simulink library "halout"  (R2021b)
settings: Solver=VariableStepAuto  StartTime=0.0  StopTime=10.0  RelTol=1e-3
undefined symbols (not defined in the file): C_TASK_5MS_S, FALSE, KHAL_CAN1FD1APS3E2E_flg, KHAL_CAN1FD1APS3TxReq_flg, KHAL_CAN1FD1VCU2E2E_flg, KHAL_CAN1FD1VCU2TxReq_flg, KHAL_CAN1FD1VCU3E2E_flg, KHAL_CAN1FD1VCU3TxReq_flg, KHAL_CAN1TxReq_flg, KHAL_CAN1VMCFCM1E2E_flg, KHAL_CAN1VMCFCM1TxReq_flg, KHAL_CAN2TxReq_flg, KHAL_CAN3FD3VCU1toNIDECTxReq_flg, KHAL_CAN3FD3VCU1TxReq_flg, KHAL_CAN3FD3VCU2E2E_flg, KHAL_CAN3FD3VCU2toNIDECE2E_flg, KHAL_CAN3FD3VCU2toNIDECTxReq_flg, KHAL_CAN3FD3VCU2TxReq_flg, KHAL_CAN3TxReq_flg, KHAL_CAN4FD4CE1000E2E_flg, KHAL_CAN4FD4CE1000TxReq_flg, KHAL_CAN4TxReq_flg, KHAL_CAN5TxReq_flg, KHAL_CAN6FD6APS3E2E_flg, KHAL_CAN6FD6APS3TxReq_flg, KHAL_CAN6FD6VCU2E2E_flg, KHAL_CAN6FD6VCU2TxReq_flg, KHAL_CAN6TxReq_flg, ONE_INT, TRUE, ZERO_INT
libraries: FVT_lib x500, simulink x235
(part 8 of 25)

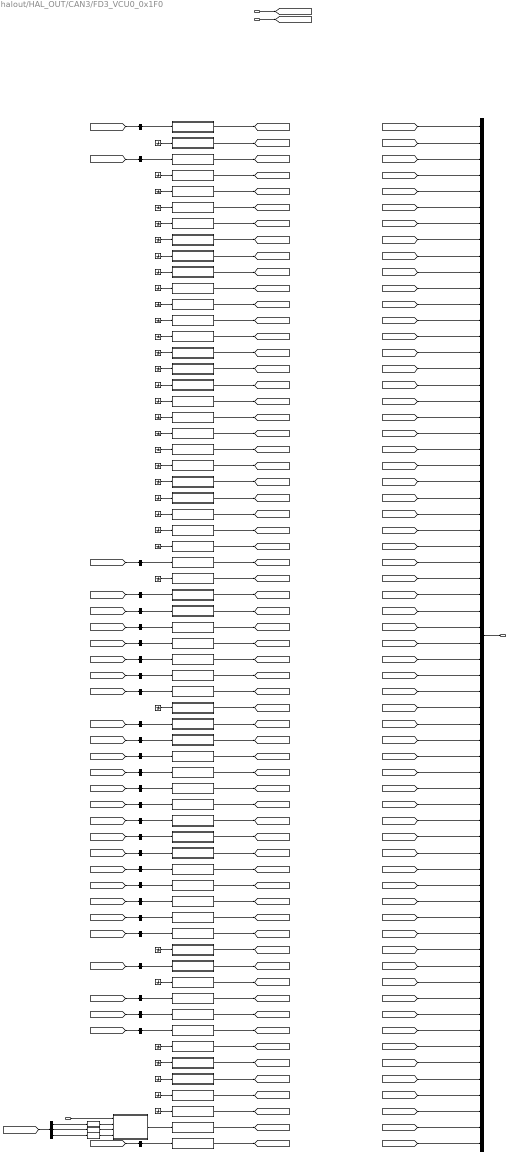
== system halout/HAL_OUT/CAN3/FD3_VCU0_0x1F0 ==
  BSCP_outputs : Inport  OutDataTypeStr=Bus: BSCP_outputs
  BOUTP_outputs : Inport  Port=2  OutDataTypeStr=Bus: BOUTP_outputs
  s8_AcoreReadyToSleep : Inport  Port=3
  Data Type Conversion : DataTypeConversion  OutDataTypeStr=uint8
  Data Type Conversion1 : DataTypeConversion  OutDataTypeStr=uint8
  Data Type Conversion2 : DataTypeConversion  OutDataTypeStr=uint8
  EVCCAplusPwrUpReq : Subsystem
  FDADC12VDet : Subsystem
  FDADC12VDetAvg : Subsystem
  FDCVCUActMaxSlideRateSta : Subsystem
  FDCVCUAllowMovThdOTASta : Subsystem
  FDCVCUDTCCarouselSta : Subsystem
  FDCVCUForcePCmd : Subsystem
  FDCVCUOTAPwrReqOFFChkSta : Subsystem
  FDCVCUOTAPwrReqStdChkSta : Subsystem
  FDCVCUPwrReqOTASta : Subsystem
  FDCVCURWDRDCActiveSta : Subsystem
  FDCVCURegenTqLimitEnSta : Subsystem
  FDCVCUSlideRegenLimTqSta : Subsystem
  FDCVCUVehActSpdSta : Subsystem
  FDCVCUVehMalfunLevelSta : Subsystem
  FDCVMCActStESCYawSta : Subsystem
  FDCVMCLongAccSta : Subsystem
  FUSIONCMM1 : Subsystem
  FUSIONCMM10 : Subsystem
  FUSIONCMM2 : Subsystem
  FUSIONCMM3 : Subsystem
  FUSIONCMM4 : Subsystem
  FUSIONCMM5 : Subsystem
  FUSIONCMM6 : Subsystem
  FUSIONCMM7 : Subsystem
  FUSIONCMM8 : Subsystem
  FUSIONCMM9 : Subsystem
  FrTqSource : Subsystem
  Ground{,1..33} (34 alike) : Ground
  HVRlyOpFail : Subsystem
  HVTHCMSysAvail : Subsystem
  LVBattChrgtimeAct : Subsystem
  LVBattVoltSta : Subsystem
  LVChrgHoldTAct : Subsystem
  LVSilentChrgLv : Subsystem
  LVSilentChrgReq : Subsystem
  LVSilentChrgSta : Subsystem
  MCUActDisFail : Subsystem
  PMMAllowECUSleep : Subsystem
  PmicBootReason : Subsystem
  PowerDownFault : Subsystem
  PowerDownState : Subsystem
  PowerUpFault : Subsystem
  PowerUpState : Subsystem
  PwrDownReq : Subsystem
  PwrStaConstraint : Subsystem
  PwrStaONTOIVIPopReq : Subsystem
  PwrStaONTOIVIPopT : Subsystem
  PwrStaSelect : Subsystem
  PwrStaTOSta : Subsystem
  PwrUpReq : Subsystem
  RrTqSource : Subsystem
  SchedChgTOSta : Subsystem
  SilentChkAllowSleep : Subsystem
  Subsystem : Subsystem
  SysAllowReadySta : Subsystem
  SysPwrSta : Subsystem
  TCountSta : Subsystem
  TimerAllowSleep : Subsystem
  VCUBrkSWSta : Subsystem
  VCUFLDoorSta : Subsystem
  VCUFRDoorSta : Subsystem
  VCURLDoorSta : Subsystem
  VCURRDoorSta : Subsystem
  VehHVPwrAvail4THCM : Subsystem
  WisrBootReason : Subsystem
  bus_creator : BusCreator  Inputs=64  OutDataTypeStr=Bus: DT_CAN3_SG_FD3_VCU0  NonVirtualBus=on
  bus_selector : BusSelector  OutputSignals=VOUTP_EvccAplusPwrUpReq_flg
  bus_selector1 : BusSelector  OutputSignals=VOUTP_FDADC12VDetAvg_mV
  bus_selector10 : BusSelector  OutputSignals=VOUTP_PMMAllowECUSleep_flg
  bus_selector11 : BusSelector  OutputSignals=VOUTP_PmicBootReason_enum
  bus_selector12 : BusSelector  OutputSignals=VOUTP_PowerDownFault_enum
  bus_selector13 : BusSelector  OutputSignals=VOUTP_PowerDownState_enum
  bus_selector14 : BusSelector  OutputSignals=VOUTP_PowerUpFault_enum
  bus_selector15 : BusSelector  OutputSignals=VOUTP_PowerUpState_enum
  bus_selector16 : BusSelector  OutputSignals=VOUTP_PwrDownReq_enum
  bus_selector17 : BusSelector  OutputSignals=VOUTP_PwrStaConstraint_enum
  bus_selector18 : BusSelector  OutputSignals=VOUTP_PwrStaONTOPopReq_flg
  bus_selector19 : BusSelector  OutputSignals=VOUTP_IVIPwrStaONTOPopT_s
  bus_selector2 : BusSelector  OutputSignals=VOUTP_TqSourceFr_enum
  bus_selector20 : BusSelector  OutputSignals=VOUTP_PwrStaSelect_enum
  bus_selector21 : BusSelector  OutputSignals=VOUTP_PwrStaTOSta_enum
  bus_selector22 : BusSelector  OutputSignals=VOUTP_PwrUpReq_enum
  bus_selector23 : BusSelector  OutputSignals=VOUTP_TqSourceRr_enum
  bus_selector24 : BusSelector  OutputSignals=VOUTP_SilentChkAllowSleep_flg
  bus_selector25 : BusSelector  OutputSignals=VOUTP_SysPowerMode_enum
  bus_selector26 : BusSelector  OutputSignals=VOUTP_TCountSta_enum
  bus_selector27 : BusSelector  OutputSignals=VOUTP_TimerAllowSleep_flg
  bus_selector28 : BusSelector  OutputSignals=VOUTP_CurrentNmState_enum,VOUTP_OTAPwrReqOFFChkSta_enum,VOUTP_OTAPwrReqStdChkSta_enum
  bus_selector29 : BusSelector  OutputSignals=VOUTP_WisrBootReason_raw32
  bus_selector3 : BusSelector  OutputSignals=VOUTP_HVTHCMSysAvail_enum
  bus_selector4 : BusSelector  OutputSignals=VOUTP_LVBattChrgTimeCnt_s
  bus_selector5 : BusSelector  OutputSignals=VOUTP_LVBattVoltSta_enum
  bus_selector6 : BusSelector  OutputSignals=VOUTP_LVChrgHoldTtimer_s
  bus_selector7 : BusSelector  OutputSignals=VOUTP_LVSilentChrgLv_enum
  bus_selector8 : BusSelector  OutputSignals=VOUTP_LVSilentChrgReq_flg
  bus_selector9 : BusSelector  OutputSignals=VOUTP_LVSilentChrgSta_enum
  FD3_VCU0 : Outport
  wires:
  BSCP_outputs/1 -> [BSCP_outputs]
  BOUTP_outputs/1 -> [BOUTP_outputs]
  [CAN3_EVCCAplusPwrUpReq] -> bus_creator/1  "CAN3_EVCCAplusPwrUpReq"
  [CAN3_FDADC12VDet] -> bus_creator/2  "CAN3_FDADC12VDet"
  [CAN3_FDADC12VDetAvg] -> bus_creator/3  "CAN3_FDADC12VDetAvg"
  [CAN3_FDC_VCU_ActMaxSlideRate_Sta] -> bus_creator/4  "CAN3_FDC_VCU_ActMaxSlideRate_Sta"
  [CAN3_FDC_VCU_AllowMovThd_OTA_Sta] -> bus_creator/5  "CAN3_FDC_VCU_AllowMovThd_OTA_Sta"
  [CAN3_FDC_VCU_DTCCarousel_Sta] -> bus_creator/6  "CAN3_FDC_VCU_DTCCarousel_Sta"
  [CAN3_FDC_VCU_ForceP_Cmd] -> bus_creator/7  "CAN3_FDC_VCU_ForceP_Cmd"
  [CAN3_FDC_VCU_OTAPwrReqOFFChk_Sta] -> bus_creator/8  "CAN3_FDC_VCU_OTAPwrReqOFFChk_Sta"
  [CAN3_FDC_VCU_OTAPwrReqStdChk_Sta] -> bus_creator/9  "CAN3_FDC_VCU_OTAPwrReqStdChk_Sta"
  [CAN3_FDC_VCU_PwrReq_OTA_Sta] -> bus_creator/10  "CAN3_FDC_VCU_PwrReq_OTA_Sta"
  [CAN3_FDC_VCU_RWDRDCActive_Sta] -> bus_creator/11  "CAN3_FDC_VCU_RWDRDCActive_Sta"
  [CAN3_FDC_VCU_RegenTqLimitEn_Sta] -> bus_creator/12  "CAN3_FDC_VCU_RegenTqLimitEn_Sta"
  [CAN3_FDC_VCU_SlideRegenLimTq_Sta] -> bus_creator/13  "CAN3_FDC_VCU_SlideRegenLimTq_Sta"
  [CAN3_FDC_VCU_VehActSpd_Sta] -> bus_creator/14  "CAN3_FDC_VCU_VehActSpd_Sta"
  [CAN3_FDC_VCU_VehMalfunLevel_Sta] -> bus_creator/15  "CAN3_FDC_VCU_VehMalfunLevel_Sta"
  [CAN3_FDC_VMC_ActStESCYaw_Sta] -> bus_creator/16  "CAN3_FDC_VMC_ActStESCYaw_Sta"
  [CAN3_FDC_VMC_LongAcc_Sta] -> bus_creator/17  "CAN3_FDC_VMC_LongAcc_Sta"
  [CAN3_FUSION_CMM1] -> bus_creator/18  "CAN3_FUSION_CMM1"
  [CAN3_FUSION_CMM10] -> bus_creator/19  "CAN3_FUSION_CMM10"
  [CAN3_FUSION_CMM2] -> bus_creator/20  "CAN3_FUSION_CMM2"
  [CAN3_FUSION_CMM3] -> bus_creator/21  "CAN3_FUSION_CMM3"
  [CAN3_FUSION_CMM4] -> bus_creator/22  "CAN3_FUSION_CMM4"
  [CAN3_FUSION_CMM5] -> bus_creator/23  "CAN3_FUSION_CMM5"
  [CAN3_FUSION_CMM6] -> bus_creator/24  "CAN3_FUSION_CMM6"
  [CAN3_FUSION_CMM7] -> bus_creator/25  "CAN3_FUSION_CMM7"
  [CAN3_FUSION_CMM8] -> bus_creator/26  "CAN3_FUSION_CMM8"
  [CAN3_FUSION_CMM9] -> bus_creator/27  "CAN3_FUSION_CMM9"
  [CAN3_Fr_TqSource] -> bus_creator/28  "CAN3_Fr_TqSource"
  [CAN3_HVRlyOpFail] -> bus_creator/29  "CAN3_HVRlyOpFail"
  [CAN3_HVTHCMSysAvail] -> bus_creator/30  "CAN3_HVTHCMSysAvail"
  [CAN3_LVBattChrgtimeAct] -> bus_creator/31  "CAN3_LVBattChrgtimeAct"
  [CAN3_LVBattVoltSta] -> bus_creator/32  "CAN3_LVBattVoltSta"
  [CAN3_LVChrgHoldTAct] -> bus_creator/33  "CAN3_LVChrgHoldTAct"
  [CAN3_LVSilentChrgLv] -> bus_creator/34  "CAN3_LVSilentChrgLv"
  [CAN3_LVSilentChrgReq] -> bus_creator/35  "CAN3_LVSilentChrgReq"
  [CAN3_LVSilentChrgSta] -> bus_creator/36  "CAN3_LVSilentChrgSta"
  [CAN3_MCUActDisFail] -> bus_creator/37  "CAN3_MCUActDisFail"
  [CAN3_PMMAllowECUSleep] -> bus_creator/38  "CAN3_PMMAllowECUSleep"
  [CAN3_PmicBootReason] -> bus_creator/39  "CAN3_PmicBootReason"
  [CAN3_PowerDownFault] -> bus_creator/40  "CAN3_PowerDownFault"
  [CAN3_PowerDownState] -> bus_creator/41  "CAN3_PowerDownState"
  [CAN3_PowerUpFault] -> bus_creator/42  "CAN3_PowerUpFault"
  [CAN3_PowerUpState] -> bus_creator/43  "CAN3_PowerUpState"
  [CAN3_PwrDownReq] -> bus_creator/44  "CAN3_PwrDownReq"
  [CAN3_PwrStaConstraint] -> bus_creator/45  "CAN3_PwrStaConstraint"
  [CAN3_PwrStaONTOIVIPopReq] -> bus_creator/46  "CAN3_PwrStaONTOIVIPopReq"
  [CAN3_PwrStaONTOIVIPopT] -> bus_creator/47  "CAN3_PwrStaONTOIVIPopT"
  [CAN3_PwrStaSelect] -> bus_creator/48  "CAN3_PwrStaSelect"
  [CAN3_PwrStaTOSta] -> bus_creator/49  "CAN3_PwrStaTOSta"
  [CAN3_PwrUpReq] -> bus_creator/50  "CAN3_PwrUpReq"
  [CAN3_Rr_TqSource] -> bus_creator/51  "CAN3_Rr_TqSource"
  [CAN3_SchedChgTOSta] -> bus_creator/52  "CAN3_SchedChgTOSta"
  [CAN3_SilentChkAllowSleep] -> bus_creator/53  "CAN3_SilentChkAllowSleep"
  [CAN3_SysAllowReadySta] -> bus_creator/54  "CAN3_SysAllowReadySta"
  [CAN3_SysPwrSta] -> bus_creator/55  "CAN3_SysPwrSta"
  [CAN3_TCountSta] -> bus_creator/56  "CAN3_TCountSta"
  [CAN3_TimerAllowSleep] -> bus_creator/57  "CAN3_TimerAllowSleep"
  [CAN3_VCUBrkSWSta] -> bus_creator/58  "CAN3_VCUBrkSWSta"
  [CAN3_VCUFLDoorSta] -> bus_creator/59  "CAN3_VCUFLDoorSta"
  [CAN3_VCUFRDoorSta] -> bus_creator/60  "CAN3_VCUFRDoorSta"
  [CAN3_VCURLDoorSta] -> bus_creator/61  "CAN3_VCURLDoorSta"
  [CAN3_VCURRDoorSta] -> bus_creator/62  "CAN3_VCURRDoorSta"
  [CAN3_VehHVPwrAvail4THCM] -> bus_creator/63  "CAN3_VehHVPwrAvail4THCM"
  [CAN3_WisrBootReason] -> bus_creator/64  "CAN3_WisrBootReason"
  bus_creator/1 -> FD3_VCU0/1
  EVCCAplusPwrUpReq/1(CAN3_EVCCAplusPwrUpReq) -> [CAN3_EVCCAplusPwrUpReq]
  FDADC12VDet/1(CAN3_FDADC12VDet) -> [CAN3_FDADC12VDet]
  FDADC12VDetAvg/1(CAN3_FDADC12VDetAvg) -> [CAN3_FDADC12VDetAvg]
  FDCVCUActMaxSlideRateSta/1(CAN3_FDC_VCU_ActMaxSlideRate_Sta) -> [CAN3_FDC_VCU_ActMaxSlideRate_Sta]
  FDCVCUAllowMovThdOTASta/1(CAN3_FDC_VCU_AllowMovThd_OTA_Sta) -> [CAN3_FDC_VCU_AllowMovThd_OTA_Sta]
  FDCVCUDTCCarouselSta/1(CAN3_FDC_VCU_DTCCarousel_Sta) -> [CAN3_FDC_VCU_DTCCarousel_Sta]
  FDCVCUForcePCmd/1(CAN3_FDC_VCU_ForceP_Cmd) -> [CAN3_FDC_VCU_ForceP_Cmd]
  FDCVCUOTAPwrReqOFFChkSta/1(CAN3_FDC_VCU_OTAPwrReqOFFChk_Sta) -> [CAN3_FDC_VCU_OTAPwrReqOFFChk_Sta]
  FDCVCUOTAPwrReqStdChkSta/1(CAN3_FDC_VCU_OTAPwrReqStdChk_Sta) -> [CAN3_FDC_VCU_OTAPwrReqStdChk_Sta]
  FDCVCUPwrReqOTASta/1(CAN3_FDC_VCU_PwrReq_OTA_Sta) -> [CAN3_FDC_VCU_PwrReq_OTA_Sta]
  FDCVCURWDRDCActiveSta/1(CAN3_FDC_VCU_RWDRDCActive_Sta) -> [CAN3_FDC_VCU_RWDRDCActive_Sta]
  FDCVCURegenTqLimitEnSta/1(CAN3_FDC_VCU_RegenTqLimitEn_Sta) -> [CAN3_FDC_VCU_RegenTqLimitEn_Sta]
  FDCVCUSlideRegenLimTqSta/1(CAN3_FDC_VCU_SlideRegenLimTq_Sta) -> [CAN3_FDC_VCU_SlideRegenLimTq_Sta]
  FDCVCUVehActSpdSta/1(CAN3_FDC_VCU_VehActSpd_Sta) -> [CAN3_FDC_VCU_VehActSpd_Sta]
  FDCVCUVehMalfunLevelSta/1(CAN3_FDC_VCU_VehMalfunLevel_Sta) -> [CAN3_FDC_VCU_VehMalfunLevel_Sta]
  FDCVMCActStESCYawSta/1(CAN3_FDC_VMC_ActStESCYaw_Sta) -> [CAN3_FDC_VMC_ActStESCYaw_Sta]
  FDCVMCLongAccSta/1(CAN3_FDC_VMC_LongAcc_Sta) -> [CAN3_FDC_VMC_LongAcc_Sta]
  FUSIONCMM1/1(CAN3_FUSION_CMM1) -> [CAN3_FUSION_CMM1]
  FUSIONCMM10/1(CAN3_FUSION_CMM10) -> [CAN3_FUSION_CMM10]
  FUSIONCMM2/1(CAN3_FUSION_CMM2) -> [CAN3_FUSION_CMM2]
  FUSIONCMM3/1(CAN3_FUSION_CMM3) -> [CAN3_FUSION_CMM3]
  FUSIONCMM4/1(CAN3_FUSION_CMM4) -> [CAN3_FUSION_CMM4]
  FUSIONCMM5/1(CAN3_FUSION_CMM5) -> [CAN3_FUSION_CMM5]
  FUSIONCMM6/1(CAN3_FUSION_CMM6) -> [CAN3_FUSION_CMM6]
  FUSIONCMM7/1(CAN3_FUSION_CMM7) -> [CAN3_FUSION_CMM7]
  FUSIONCMM8/1(CAN3_FUSION_CMM8) -> [CAN3_FUSION_CMM8]
  FUSIONCMM9/1(CAN3_FUSION_CMM9) -> [CAN3_FUSION_CMM9]
  FrTqSource/1(CAN3_Fr_TqSource) -> [CAN3_Fr_TqSource]
  HVRlyOpFail/1(CAN3_HVRlyOpFail) -> [CAN3_HVRlyOpFail]
  HVTHCMSysAvail/1(CAN3_HVTHCMSysAvail) -> [CAN3_HVTHCMSysAvail]
  LVBattChrgtimeAct/1(CAN3_LVBattChrgtimeAct) -> [CAN3_LVBattChrgtimeAct]
  LVBattVoltSta/1(CAN3_LVBattVoltSta) -> [CAN3_LVBattVoltSta]
  LVChrgHoldTAct/1(CAN3_LVChrgHoldTAct) -> [CAN3_LVChrgHoldTAct]
  LVSilentChrgLv/1(CAN3_LVSilentChrgLv) -> [CAN3_LVSilentChrgLv]
  LVSilentChrgReq/1(CAN3_LVSilentChrgReq) -> [CAN3_LVSilentChrgReq]
  LVSilentChrgSta/1(CAN3_LVSilentChrgSta) -> [CAN3_LVSilentChrgSta]
  MCUActDisFail/1(CAN3_MCUActDisFail) -> [CAN3_MCUActDisFail]
  PMMAllowECUSleep/1(CAN3_PMMAllowECUSleep) -> [CAN3_PMMAllowECUSleep]
  PmicBootReason/1(CAN3_PmicBootReason) -> [CAN3_PmicBootReason]
  PowerDownFault/1(CAN3_PowerDownFault) -> [CAN3_PowerDownFault]
  PowerDownState/1(CAN3_PowerDownState) -> [CAN3_PowerDownState]
  PowerUpFault/1(CAN3_PowerUpFault) -> [CAN3_PowerUpFault]
  PowerUpState/1(CAN3_PowerUpState) -> [CAN3_PowerUpState]
  PwrDownReq/1(CAN3_PwrDownReq) -> [CAN3_PwrDownReq]
  PwrStaConstraint/1(CAN3_PwrStaConstraint) -> [CAN3_PwrStaConstraint]
  PwrStaONTOIVIPopReq/1(CAN3_PwrStaONTOIVIPopReq) -> [CAN3_PwrStaONTOIVIPopReq]
  PwrStaONTOIVIPopT/1(CAN3_PwrStaONTOIVIPopT) -> [CAN3_PwrStaONTOIVIPopT]
  PwrStaSelect/1(CAN3_PwrStaSelect) -> [CAN3_PwrStaSelect]
  PwrStaTOSta/1(CAN3_PwrStaTOSta) -> [CAN3_PwrStaTOSta]
  PwrUpReq/1(CAN3_PwrUpReq) -> [CAN3_PwrUpReq]
  RrTqSource/1(CAN3_Rr_TqSource) -> [CAN3_Rr_TqSource]
  SchedChgTOSta/1(CAN3_SchedChgTOSta) -> [CAN3_SchedChgTOSta]
  SilentChkAllowSleep/1(CAN3_SilentChkAllowSleep) -> [CAN3_SilentChkAllowSleep]
  SysAllowReadySta/1(CAN3_SysAllowReadySta) -> [CAN3_SysAllowReadySta]
  SysPwrSta/1(CAN3_SysPwrSta) -> [CAN3_SysPwrSta]
  TCountSta/1(CAN3_TCountSta) -> [CAN3_TCountSta]
  TimerAllowSleep/1(CAN3_TimerAllowSleep) -> [CAN3_TimerAllowSleep]
  VCUBrkSWSta/1(CAN3_VCUBrkSWSta) -> [CAN3_VCUBrkSWSta]
  VCUFLDoorSta/1(CAN3_VCUFLDoorSta) -> [CAN3_VCUFLDoorSta]
  VCUFRDoorSta/1(CAN3_VCUFRDoorSta) -> [CAN3_VCUFRDoorSta]
  VCURLDoorSta/1(CAN3_VCURLDoorSta) -> [CAN3_VCURLDoorSta]
  VCURRDoorSta/1(CAN3_VCURRDoorSta) -> [CAN3_VCURRDoorSta]
  VehHVPwrAvail4THCM/1(CAN3_VehHVPwrAvail4THCM) -> [CAN3_VehHVPwrAvail4THCM]
  WisrBootReason/1(CAN3_WisrBootReason) -> [CAN3_WisrBootReason]
  bus_selector/1 -> EVCCAplusPwrUpReq/1(EVCCAplusPwrUpReq)  "<VOUTP_EvccAplusPwrUpReq_flg>"
  [BOUTP_outputs] -> bus_selector/1
  Ground/1 -> FDADC12VDet/1(FDADC12VDet)
  bus_selector1/1 -> FDADC12VDetAvg/1(FDADC12VDetAvg)  "<VOUTP_FDADC12VDetAvg_mV>"
  [BOUTP_outputs] -> bus_selector1/1
  Ground1/1 -> FDCVCUActMaxSlideRateSta/1(FDCVCUActMaxSlideRateSta)
  Ground2/1 -> FDCVCUAllowMovThdOTASta/1(FDCVCUAllowMovThdOTASta)
  Ground3/1 -> FDCVCUDTCCarouselSta/1(FDCVCUDTCCarouselSta)
  Ground4/1 -> FDCVCUForcePCmd/1(FDCVCUForcePCmd)
  Ground5/1 -> FDCVCUOTAPwrReqOFFChkSta/1(FDCVCUOTAPwrReqOFFChkSta)
  Ground6/1 -> FDCVCUOTAPwrReqStdChkSta/1(FDCVCUOTAPwrReqStdChkSta)
  Ground7/1 -> FDCVCUPwrReqOTASta/1(FDCVCUPwrReqOTASta)
  Ground8/1 -> FDCVCURWDRDCActiveSta/1(FDCVCURWDRDCActiveSta)
  Ground9/1 -> FDCVCURegenTqLimitEnSta/1(FDCVCURegenTqLimitEnSta)
  Ground10/1 -> FDCVCUSlideRegenLimTqSta/1(FDCVCUSlideRegenLimTqSta)
  Ground11/1 -> FDCVCUVehActSpdSta/1(FDCVCUVehActSpdSta)
  Ground12/1 -> FDCVCUVehMalfunLevelSta/1(FDCVCUVehMalfunLevelSta)
  Ground13/1 -> FDCVMCActStESCYawSta/1(FDCVMCActStESCYawSta)
  Ground14/1 -> FDCVMCLongAccSta/1(FDCVMCLongAccSta)
  Ground15/1 -> FUSIONCMM1/1(FUSIONCMM1)
  Ground16/1 -> FUSIONCMM10/1(FUSIONCMM10)
  Ground17/1 -> FUSIONCMM2/1(FUSIONCMM2)
  Ground18/1 -> FUSIONCMM3/1(FUSIONCMM3)
  Ground19/1 -> FUSIONCMM4/1(FUSIONCMM4)
  Ground20/1 -> FUSIONCMM5/1(FUSIONCMM5)
  Ground21/1 -> FUSIONCMM6/1(FUSIONCMM6)
  Ground22/1 -> FUSIONCMM7/1(FUSIONCMM7)
  Ground23/1 -> FUSIONCMM8/1(FUSIONCMM8)
  Ground24/1 -> FUSIONCMM9/1(FUSIONCMM9)
  bus_selector2/1 -> FrTqSource/1(FrTqSource)  "<VOUTP_TqSourceFr_enum>"
  [BOUTP_outputs] -> bus_selector2/1
  Ground25/1 -> HVRlyOpFail/1(HVRlyOpFail)
  bus_selector3/1 -> HVTHCMSysAvail/1(HVTHCMSysAvail)  "<VOUTP_HVTHCMSysAvail_enum>"
  [BOUTP_outputs] -> bus_selector3/1
  bus_selector4/1 -> LVBattChrgtimeAct/1(LVBattChrgtimeAct)  "<VOUTP_LVBattChrgTimeCnt_s>"
  [BOUTP_outputs] -> bus_selector4/1
  bus_selector5/1 -> LVBattVoltSta/1(LVBattVoltSta)  "<VOUTP_LVBattVoltSta_enum>"
  [BOUTP_outputs] -> bus_selector5/1
  bus_selector6/1 -> LVChrgHoldTAct/1(LVChrgHoldTAct)  "<VOUTP_LVChrgHoldTtimer_s>"
  [BOUTP_outputs] -> bus_selector6/1
  bus_selector7/1 -> LVSilentChrgLv/1(LVSilentChrgLv)  "<VOUTP_LVSilentChrgLv_enum>"
  [BOUTP_outputs] -> bus_selector7/1
  bus_selector8/1 -> LVSilentChrgReq/1(LVSilentChrgReq)  "<VOUTP_LVSilentChrgReq_flg>"
  [BOUTP_outputs] -> bus_selector8/1
  bus_selector9/1 -> LVSilentChrgSta/1(LVSilentChrgSta)  "<VOUTP_LVSilentChrgSta_enum>"
  [BOUTP_outputs] -> bus_selector9/1
  Ground26/1 -> MCUActDisFail/1(MCUActDisFail)
  bus_selector10/1 -> PMMAllowECUSleep/1(PMMAllowECUSleep)  "<VOUTP_PMMAllowECUSleep_flg>"
  [BOUTP_outputs] -> bus_selector10/1
  bus_selector11/1 -> PmicBootReason/1(PmicBootReason)  "<VOUTP_PmicBootReason_enum>"
  [BOUTP_outputs] -> bus_selector11/1
  bus_selector12/1 -> PowerDownFault/1(PowerDownFault)  "<VOUTP_PowerDownFault_enum>"
  [BOUTP_outputs] -> bus_selector12/1
  bus_selector13/1 -> PowerDownState/1(PowerDownState)  "<VOUTP_PowerDownState_enum>"
  [BOUTP_outputs] -> bus_selector13/1
  bus_selector14/1 -> PowerUpFault/1(PowerUpFault)  "<VOUTP_PowerUpFault_enum>"
  [BOUTP_outputs] -> bus_selector14/1
  bus_selector15/1 -> PowerUpState/1(PowerUpState)  "<VOUTP_PowerUpState_enum>"
  [BOUTP_outputs] -> bus_selector15/1
  bus_selector16/1 -> PwrDownReq/1(PwrDownReq)  "<VOUTP_PwrDownReq_enum>"
  [BOUTP_outputs] -> bus_selector16/1
  bus_selector17/1 -> PwrStaConstraint/1(PwrStaConstraint)  "<VOUTP_PwrStaConstraint_enum>"
  [BOUTP_outputs] -> bus_selector17/1
  bus_selector18/1 -> PwrStaONTOIVIPopReq/1(PwrStaONTOIVIPopReq)  "<VOUTP_PwrStaONTOPopReq_flg>"
  [BOUTP_outputs] -> bus_selector18/1
  bus_selector19/1 -> PwrStaONTOIVIPopT/1(PwrStaONTOIVIPopT)  "<VOUTP_IVIPwrStaONTOPopT_s>"
  [BOUTP_outputs] -> bus_selector19/1
  bus_selector20/1 -> PwrStaSelect/1(PwrStaSelect)  "<VOUTP_PwrStaSelect_enum>"
  [BOUTP_outputs] -> bus_selector20/1
  bus_selector21/1 -> PwrStaTOSta/1(PwrStaTOSta)  "<VOUTP_PwrStaTOSta_enum>"
  [BOUTP_outputs] -> bus_selector21/1
  bus_selector22/1 -> PwrUpReq/1(PwrUpReq)  "<VOUTP_PwrUpReq_enum>"
  [BOUTP_outputs] -> bus_selector22/1
  bus_selector23/1 -> RrTqSource/1(RrTqSource)  "<VOUTP_TqSourceRr_enum>"
  [BOUTP_outputs] -> bus_selector23/1
  Ground27/1 -> SchedChgTOSta/1(SchedChgTOSta)
  bus_selector24/1 -> SilentChkAllowSleep/1(SilentChkAllowSleep)  "<VOUTP_SilentChkAllowSleep_flg>"
  [BOUTP_outputs] -> bus_selector24/1
  Ground28/1 -> SysAllowReadySta/1(SysAllowReadySta)
  bus_selector25/1 -> SysPwrSta/1(SysPwrSta)  "<VOUTP_SysPowerMode_enum>"
  [BOUTP_outputs] -> bus_selector25/1
  bus_selector26/1 -> TCountSta/1(TCountSta)  "<VOUTP_TCountSta_enum>"
  [BOUTP_outputs] -> bus_selector26/1
  bus_selector27/1 -> TimerAllowSleep/1(TimerAllowSleep)  "<VOUTP_TimerAllowSleep_flg>"
  [BOUTP_outputs] -> bus_selector27/1
  Ground29/1 -> VCUBrkSWSta/1(VCUBrkSWSta)
  Ground30/1 -> VCUFLDoorSta/1(VCUFLDoorSta)
  Ground31/1 -> VCUFRDoorSta/1(VCUFRDoorSta)
  Ground32/1 -> VCURLDoorSta/1(VCURLDoorSta)
  Ground33/1 -> VCURRDoorSta/1(VCURRDoorSta)
  bus_selector29/1 -> WisrBootReason/1(WisrBootReason)  "<VOUTP_WisrBootReason_raw32>"
  [BOUTP_outputs] -> bus_selector29/1
  Subsystem/1(VehHVPwrAvail4THCM) -> VehHVPwrAvail4THCM/1(VehHVPwrAvail4THCM)
  bus_selector28/2 -> Data Type Conversion1/1  "<VOUTP_OTAPwrReqOFFChkSta_enum>"
  Data Type Conversion2/1 -> Subsystem/4(VOUTP_OTAPwrReqStdChkSta_enum)
  bus_selector28/1 -> Data Type Conversion/1  "<VOUTP_CurrentNmState_enum>"
  bus_selector28/3 -> Data Type Conversion2/1  "<VOUTP_OTAPwrReqStdChkSta_enum>"
  Data Type Conversion1/1 -> Subsystem/3(VOUTP_OTAPwrReqOFFChkSta_enum)
  Data Type Conversion/1 -> Subsystem/2(VOUTP_CurrentNmState_enum)
  [BOUTP_outputs] -> bus_selector28/1
  s8_AcoreReadyToSleep/1 -> Subsystem/1(s8_AcoreReadyToSleep)

== system halout/HAL_OUT/CAN3/FD3_VCU1_0x115 ==
  BSCP_outputs : Inport  OutDataTypeStr=Bus: BSCP_outputs
  BOUTP_outputs : Inport  Port=2  OutDataTypeStr=Bus: BOUTP_outputs
  ActiveDischReq : Subsystem
  CSVCU1 : Subsystem
  CoastDwModeStaChk : Subsystem
  DCDCEnaReq : Subsystem
  DCDCVoltSetpoint : Subsystem
  DemoModeStaChk : Subsystem
  DrSeatSta : Subsystem
  DynoModeStaChk : Subsystem
  Ground{,1..6} (7 alike) : Ground
  HVBatCnctReq : Subsystem
  HVSysReadyToCharge : Subsystem
  LVChrgFuncStaChk : Subsystem
  MSACrlSta : Subsystem
  PButtonSta : Subsystem
  PrkReq : Subsystem
  PrkReqValid : Subsystem
  PwrSta : Subsystem
  RCVCU1 : Subsystem
  ShiftGearPosn : Subsystem
  bus_creator : BusCreator  Inputs=18  OutDataTypeStr=Bus: DT_CAN3_SG_FD3_VCU1  NonVirtualBus=on
  bus_selector : BusSelector  OutputSignals=VOUTP_ActiveDischargeReq_flg
  bus_selector1 : BusSelector  OutputSignals=VOUTP_DCDCEnaReq_flg
  bus_selector10 : BusSelector  OutputSignals=VOUTP_ShiftGearPosn_enum
  bus_selector2 : BusSelector  OutputSignals=VOUTP_DCDCVoltSetpoint_V
  bus_selector3 : BusSelector  OutputSignals=VOUTP_DrSeatSta_enum
  bus_selector4 : BusSelector  OutputSignals=VOUTP_HVBatCnctReq_flg
  bus_selector5 : BusSelector  OutputSignals=VOUTP_HVSysReadyToCharge_enum
  bus_selector6 : BusSelector  OutputSignals=VOUTP_MSACtrlSta_enum
  bus_selector7 : BusSelector  OutputSignals=VOUTP_PButtonSta_enum
  bus_selector8 : BusSelector  OutputSignals=VOUTP_ActParkRequest_flg
  bus_selector9 : BusSelector  OutputSignals=VOUTP_PowerSta_enum
  FD3_VCU1 : Outport
  wires:
  BSCP_outputs/1 -> [BSCP_outputs]
  BOUTP_outputs/1 -> [BOUTP_outputs]
  [CAN3_ActiveDischReq] -> bus_creator/1  "CAN3_ActiveDischReq"
  [CAN3_CS_VCU1] -> bus_creator/2  "CAN3_CS_VCU1"
  [CAN3_CoastDwModeStaChk] -> bus_creator/3  "CAN3_CoastDwModeStaChk"
  [CAN3_DCDCEnaReq] -> bus_creator/4  "CAN3_DCDCEnaReq"
  [CAN3_DCDCVoltSetpoint] -> bus_creator/5  "CAN3_DCDCVoltSetpoint"
  [CAN3_DemoModeStaChk] -> bus_creator/6  "CAN3_DemoModeStaChk"
  [CAN3_Dr_SeatSta] -> bus_creator/7  "CAN3_Dr_SeatSta"
  [CAN3_DynoModeStaChk] -> bus_creator/8  "CAN3_DynoModeStaChk"
  [CAN3_HVBatCnctReq] -> bus_creator/9  "CAN3_HVBatCnctReq"
  [CAN3_HVSysReadyToCharge] -> bus_creator/10  "CAN3_HVSysReadyToCharge"
  [CAN3_LVChrgFuncStaChk] -> bus_creator/11  "CAN3_LVChrgFuncStaChk"
  [CAN3_MSA_Crl_Sta] -> bus_creator/12  "CAN3_MSA_Crl_Sta"
  [CAN3_P_Button_Sta] -> bus_creator/13  "CAN3_P_Button_Sta"
  [CAN3_PrkReq] -> bus_creator/14  "CAN3_PrkReq"
  [CAN3_PrkReqValid] -> bus_creator/15  "CAN3_PrkReqValid"
  [CAN3_PwrSta] -> bus_creator/16  "CAN3_PwrSta"
  [CAN3_RC_VCU1] -> bus_creator/17  "CAN3_RC_VCU1"
  [CAN3_ShiftGearPosn] -> bus_creator/18  "CAN3_ShiftGearPosn"
  bus_creator/1 -> FD3_VCU1/1
  ActiveDischReq/1(CAN3_ActiveDischReq) -> [CAN3_ActiveDischReq]
  CSVCU1/1(CAN3_CS_VCU1) -> [CAN3_CS_VCU1]
  CoastDwModeStaChk/1(CAN3_CoastDwModeStaChk) -> [CAN3_CoastDwModeStaChk]
  DCDCEnaReq/1(CAN3_DCDCEnaReq) -> [CAN3_DCDCEnaReq]
  DCDCVoltSetpoint/1(CAN3_DCDCVoltSetpoint) -> [CAN3_DCDCVoltSetpoint]
  DemoModeStaChk/1(CAN3_DemoModeStaChk) -> [CAN3_DemoModeStaChk]
  DrSeatSta/1(CAN3_Dr_SeatSta) -> [CAN3_Dr_SeatSta]
  DynoModeStaChk/1(CAN3_DynoModeStaChk) -> [CAN3_DynoModeStaChk]
  HVBatCnctReq/1(CAN3_HVBatCnctReq) -> [CAN3_HVBatCnctReq]
  HVSysReadyToCharge/1(CAN3_HVSysReadyToCharge) -> [CAN3_HVSysReadyToCharge]
  LVChrgFuncStaChk/1(CAN3_LVChrgFuncStaChk) -> [CAN3_LVChrgFuncStaChk]
  MSACrlSta/1(CAN3_MSA_Crl_Sta) -> [CAN3_MSA_Crl_Sta]
  PButtonSta/1(CAN3_P_Button_Sta) -> [CAN3_P_Button_Sta]
  PrkReq/1(CAN3_PrkReq) -> [CAN3_PrkReq]
  PrkReqValid/1(CAN3_PrkReqValid) -> [CAN3_PrkReqValid]
  PwrSta/1(CAN3_PwrSta) -> [CAN3_PwrSta]
  RCVCU1/1(CAN3_RC_VCU1) -> [CAN3_RC_VCU1]
  ShiftGearPosn/1(CAN3_ShiftGearPosn) -> [CAN3_ShiftGearPosn]
  bus_selector/1 -> ActiveDischReq/1(ActiveDischReq)  "<VOUTP_ActiveDischargeReq_flg>"
  [BOUTP_outputs] -> bus_selector/1
  Ground/1 -> CSVCU1/1(CSVCU1)
  Ground1/1 -> CoastDwModeStaChk/1(CoastDwModeStaChk)
  bus_selector1/1 -> DCDCEnaReq/1(DCDCEnaReq)  "<VOUTP_DCDCEnaReq_flg>"
  [BOUTP_outputs] -> bus_selector1/1
  bus_selector2/1 -> DCDCVoltSetpoint/1(DCDCVoltSetpoint)  "<VOUTP_DCDCVoltSetpoint_V>"
  [BOUTP_outputs] -> bus_selector2/1
  Ground2/1 -> DemoModeStaChk/1(DemoModeStaChk)
  bus_selector3/1 -> DrSeatSta/1(DrSeatSta)  "<VOUTP_DrSeatSta_enum>"
  [BOUTP_outputs] -> bus_selector3/1
  Ground3/1 -> DynoModeStaChk/1(DynoModeStaChk)
  bus_selector4/1 -> HVBatCnctReq/1(HVBatCnctReq)  "<VOUTP_HVBatCnctReq_flg>"
  [BOUTP_outputs] -> bus_selector4/1
  bus_selector5/1 -> HVSysReadyToCharge/1(HVSysReadyToCharge)  "<VOUTP_HVSysReadyToCharge_enum>"
  [BOUTP_outputs] -> bus_selector5/1
  Ground4/1 -> LVChrgFuncStaChk/1(LVChrgFuncStaChk)
  bus_selector6/1 -> MSACrlSta/1(MSACrlSta)  "<VOUTP_MSACtrlSta_enum>"
  [BOUTP_outputs] -> bus_selector6/1
  bus_selector7/1 -> PButtonSta/1(PButtonSta)  "<VOUTP_PButtonSta_enum>"
  [BOUTP_outputs] -> bus_selector7/1
  bus_selector8/1 -> PrkReq/1(PrkReq)  "<VOUTP_ActParkRequest_flg>"
  [BOUTP_outputs] -> bus_selector8/1
  Ground5/1 -> PrkReqValid/1(PrkReqValid)
  bus_selector9/1 -> PwrSta/1(PwrSta)  "<VOUTP_PowerSta_enum>"
  [BOUTP_outputs] -> bus_selector9/1
  Ground6/1 -> RCVCU1/1(RCVCU1)
  bus_selector10/1 -> ShiftGearPosn/1(ShiftGearPosn)  "<VOUTP_ShiftGearPosn_enum>"
  [BOUTP_outputs] -> bus_selector10/1

== system halout/HAL_OUT/CAN3/FD3_VCU1_Tx ==
  TxReq : Inport
  BSCP_outputs : Inport  Port=2  OutDataTypeStr=Bus: BSCP_outputs
  BOUTP_outputs : Inport  Port=3  OutDataTypeStr=Bus: BOUTP_outputs
  Chart : Stateflow chart  TreatAsAtomicUnit=on
  Constant : Constant  Value=C_TASK_5MS_S
  Constant3 : Constant  Value=CycleTime
  Data Type Conversion : DataTypeConversion  OutDataTypeStr=uint16
  Data Type Conversion1 : DataTypeConversion  OutDataTypeStr=uint8
  Divide : Product  Inputs=*/
  Gain : Gain  Gain=0.001
  Ground{,1..6} (7 alike) : Ground
  OR : Logic  Operator=OR  Inputs=18  AllPortsSameDT=off  OutDataTypeStr=boolean
  bus_selector : BusSelector  OutputSignals=VOUTP_ActiveDischargeReq_flg
  bus_selector1 : BusSelector  OutputSignals=VOUTP_DCDCEnaReq_flg
  bus_selector10 : BusSelector  OutputSignals=VOUTP_ShiftGearPosn_enum
  bus_selector2 : BusSelector  OutputSignals=VOUTP_DCDCVoltSetpoint_V
  bus_selector3 : BusSelector  OutputSignals=VOUTP_DrSeatSta_enum
  bus_selector4 : BusSelector  OutputSignals=VOUTP_HVBatCnctReq_flg
  bus_selector5 : BusSelector  OutputSignals=VOUTP_HVSysReadyToCharge_enum
  bus_selector6 : BusSelector  OutputSignals=VOUTP_MSACtrlSta_enum
  bus_selector7 : BusSelector  OutputSignals=VOUTP_PButtonSta_enum
  bus_selector8 : BusSelector  OutputSignals=VOUTP_ActParkRequest_flg
  bus_selector9 : BusSelector  OutputSignals=VOUTP_PowerSta_enum
  convert_out : FVT_lib/hal/convert_out  gain=0.0235  offset=12
  detect_change{,1..10} (11 alike) : simulink/Logic and Bit Operations/Detect Change  vinit=0  OutDataTypeStr=boolean
  TxTrigger : Outport
  wires:
  Data Type Conversion/1 -> Chart/3(CycleCnt)
  TxReq/1 -> Chart/1(TxReq)
  [EventReq_flg] -> Chart/2(EventReq)
  Constant/1 -> Divide/2
  Divide/1 -> Data Type Conversion/1
  Chart/1(TxTrigger) -> TxTrigger/1
  Gain/1 -> Divide/1
  Constant3/1 -> Gain/1
  BSCP_outputs/1 -> [BSCP_outputs]
  BOUTP_outputs/1 -> [BOUTP_outputs]
  OR/1 -> [EventReq_flg]
  detect_change/1 -> OR/1
  bus_selector/1 -> detect_change/1  "<VOUTP_ActiveDischargeReq_flg>"
  [BOUTP_outputs] -> bus_selector/1
  Ground/1 -> OR/2
  Ground1/1 -> OR/3
  detect_change1/1 -> OR/4
  bus_selector1/1 -> detect_change1/1  "<VOUTP_DCDCEnaReq_flg>"
  [BOUTP_outputs] -> bus_selector1/1
  detect_change2/1 -> OR/5
  Data Type Conversion1/1 -> detect_change2/1
  convert_out/1 -> Data Type Conversion1/1
  bus_selector2/1 -> convert_out/1  "<VOUTP_DCDCVoltSetpoint_V>"
  [BOUTP_outputs] -> bus_selector2/1
  Ground2/1 -> OR/6
  detect_change3/1 -> OR/7
  bus_selector3/1 -> detect_change3/1  "<VOUTP_DrSeatSta_enum>"
  [BOUTP_outputs] -> bus_selector3/1
  Ground3/1 -> OR/8
  detect_change4/1 -> OR/9
  bus_selector4/1 -> detect_change4/1  "<VOUTP_HVBatCnctReq_flg>"
  [BOUTP_outputs] -> bus_selector4/1
  detect_change5/1 -> OR/10
  bus_selector5/1 -> detect_change5/1  "<VOUTP_HVSysReadyToCharge_enum>"
  [BOUTP_outputs] -> bus_selector5/1
  Ground4/1 -> OR/11
  detect_change6/1 -> OR/12
  bus_selector6/1 -> detect_change6/1  "<VOUTP_MSACtrlSta_enum>"
  [BOUTP_outputs] -> bus_selector6/1
  detect_change7/1 -> OR/13
  bus_selector7/1 -> detect_change7/1  "<VOUTP_PButtonSta_enum>"
  [BOUTP_outputs] -> bus_selector7/1
  detect_change8/1 -> OR/14
  bus_selector8/1 -> detect_change8/1  "<VOUTP_ActParkRequest_flg>"
  [BOUTP_outputs] -> bus_selector8/1
  Ground5/1 -> OR/15
  detect_change9/1 -> OR/16
  bus_selector9/1 -> detect_change9/1  "<VOUTP_PowerSta_enum>"
  [BOUTP_outputs] -> bus_selector9/1
  Ground6/1 -> OR/17
  detect_change10/1 -> OR/18
  bus_selector10/1 -> detect_change10/1  "<VOUTP_ShiftGearPosn_enum>"
  [BOUTP_outputs] -> bus_selector10/1

== system halout/HAL_OUT/CAN3/FD3_VCU1_toNIDEC_0x116 ==
  BSCP_outputs : Inport  OutDataTypeStr=Bus: BSCP_outputs
  BOUTP_outputs : Inport  Port=2  OutDataTypeStr=Bus: BOUTP_outputs
  ActiveDischReqtoNidec : Subsystem
  CSVCU1toNidec : Subsystem
  CoastDwModeStaChktoNidec : Subsystem
  DCDCEnaReqtoNidec : Subsystem
  DCDCVoltSetpointtoNidec : Subsystem
  DemoModeStaChktoNidec : Subsystem
  DrSeatStatoNidec : Subsystem
  DynoModeStaChktoNidec : Subsystem
  FrActvDmpDisabReqtoNidec : Subsystem
  FrMCUEnaReqtoNidec : Subsystem
  Ground{,1..5} (6 alike) : Ground
  HVBatCnctReqtoNidec : Subsystem
  HVSysReadyToChargetoNidec : Subsystem
  LVChrgFuncStaChktoNidec : Subsystem
  MSACrlStatoNidec : Subsystem
  PrkReqtoNidec : Subsystem
  PwrStatoNidec : Subsystem
  RCVCU1toNidec : Subsystem
  RrActvDmpDisabReqtoNidec : Subsystem
  RrMCUEnaReqtoNidec : Subsystem
  ShiftGearPosntoNidec : Subsystem
  bus_creator : BusCreator  Inputs=20  OutDataTypeStr=Bus: DT_CAN3_SG_FD3_VCU1_toNIDEC  NonVirtualBus=on
  bus_selector : BusSelector  OutputSignals=VOUTP_ActiveDischargeReq_flg
  bus_selector1 : BusSelector  OutputSignals=VOUTP_DCDCEnaReq_flg
  bus_selector10 : BusSelector  OutputSignals=VOUTP_PowerSta_enum
  bus_selector11 : BusSelector  OutputSignals=VOUTP_RrActvDmpDisabReq_flg
  bus_selector12 : BusSelector  OutputSignals=VOUTP_RrMCUEnaReq_flg
  bus_selector13 : BusSelector  OutputSignals=VOUTP_ShiftGearPosn_enum
  bus_selector2 : BusSelector  OutputSignals=VOUTP_DCDCVoltSetpoint_V
  bus_selector3 : BusSelector  OutputSignals=VOUTP_DrSeatSta_enum
  bus_selector4 : BusSelector  OutputSignals=VOUTP_FrActvDmpDisabReq_flg
  bus_selector5 : BusSelector  OutputSignals=VOUTP_FrMCUEnaReq_flg
  bus_selector6 : BusSelector  OutputSignals=VOUTP_HVBatCnctReq_flg
  bus_selector7 : BusSelector  OutputSignals=VOUTP_HVSysReadyToCharge_enum
  bus_selector8 : BusSelector  OutputSignals=VOUTP_MSACtrlSta_enum
  bus_selector9 : BusSelector  OutputSignals=VOUTP_ActParkRequest_flg
  FD3_VCU1_toNIDEC : Outport
  wires:
  BSCP_outputs/1 -> [BSCP_outputs]
  BOUTP_outputs/1 -> [BOUTP_outputs]
  [CAN3_ActiveDischReq_toNidec] -> bus_creator/1  "CAN3_ActiveDischReq_toNidec"
  [CAN3_CS_VCU1_toNidec] -> bus_creator/2  "CAN3_CS_VCU1_toNidec"
  [CAN3_CoastDwModeStaChk_toNidec] -> bus_creator/3  "CAN3_CoastDwModeStaChk_toNidec"
  [CAN3_DCDCEnaReq_toNidec] -> bus_creator/4  "CAN3_DCDCEnaReq_toNidec"
  [CAN3_DCDCVoltSetpoint_toNidec] -> bus_creator/5  "CAN3_DCDCVoltSetpoint_toNidec"
  [CAN3_DemoModeStaChk_toNidec] -> bus_creator/6  "CAN3_DemoModeStaChk_toNidec"
  [CAN3_Dr_SeatSta_toNidec] -> bus_creator/7  "CAN3_Dr_SeatSta_toNidec"
  [CAN3_DynoModeStaChk_toNidec] -> bus_creator/8  "CAN3_DynoModeStaChk_toNidec"
  [CAN3_Fr_ActvDmpDisabReq_toNidec] -> bus_creator/9  "CAN3_Fr_ActvDmpDisabReq_toNidec"
  [CAN3_Fr_MCUEnaReq_toNidec] -> bus_creator/10  "CAN3_Fr_MCUEnaReq_toNidec"
  [CAN3_HVBatCnctReq_toNidec] -> bus_creator/11  "CAN3_HVBatCnctReq_toNidec"
  [CAN3_HVSysReadyToCharge_toNidec] -> bus_creator/12  "CAN3_HVSysReadyToCharge_toNidec"
  [CAN3_LVChrgFuncStaChk_toNidec] -> bus_creator/13  "CAN3_LVChrgFuncStaChk_toNidec"
  [CAN3_MSA_Crl_Sta_toNidec] -> bus_creator/14  "CAN3_MSA_Crl_Sta_toNidec"
  [CAN3_PrkReq_toNidec] -> bus_creator/15  "CAN3_PrkReq_toNidec"
  [CAN3_PwrSta_toNidec] -> bus_creator/16  "CAN3_PwrSta_toNidec"
  [CAN3_RC_VCU1_toNidec] -> bus_creator/17  "CAN3_RC_VCU1_toNidec"
  [CAN3_Rr_ActvDmpDisabReq_toNidec] -> bus_creator/18  "CAN3_Rr_ActvDmpDisabReq_toNidec"
  [CAN3_Rr_MCUEnaReq_toNidec] -> bus_creator/19  "CAN3_Rr_MCUEnaReq_toNidec"
  [CAN3_ShiftGearPosn_toNidec] -> bus_creator/20  "CAN3_ShiftGearPosn_toNidec"
  bus_creator/1 -> FD3_VCU1_toNIDEC/1
  ActiveDischReqtoNidec/1(CAN3_ActiveDischReq_toNidec) -> [CAN3_ActiveDischReq_toNidec]
  CSVCU1toNidec/1(CAN3_CS_VCU1_toNidec) -> [CAN3_CS_VCU1_toNidec]
  CoastDwModeStaChktoNidec/1(CAN3_CoastDwModeStaChk_toNidec) -> [CAN3_CoastDwModeStaChk_toNidec]
  DCDCEnaReqtoNidec/1(CAN3_DCDCEnaReq_toNidec) -> [CAN3_DCDCEnaReq_toNidec]
  DCDCVoltSetpointtoNidec/1(CAN3_DCDCVoltSetpoint_toNidec) -> [CAN3_DCDCVoltSetpoint_toNidec]
  DemoModeStaChktoNidec/1(CAN3_DemoModeStaChk_toNidec) -> [CAN3_DemoModeStaChk_toNidec]
  DrSeatStatoNidec/1(CAN3_Dr_SeatSta_toNidec) -> [CAN3_Dr_SeatSta_toNidec]
  DynoModeStaChktoNidec/1(CAN3_DynoModeStaChk_toNidec) -> [CAN3_DynoModeStaChk_toNidec]
  FrActvDmpDisabReqtoNidec/1(CAN3_Fr_ActvDmpDisabReq_toNidec) -> [CAN3_Fr_ActvDmpDisabReq_toNidec]
  FrMCUEnaReqtoNidec/1(CAN3_Fr_MCUEnaReq_toNidec) -> [CAN3_Fr_MCUEnaReq_toNidec]
  HVBatCnctReqtoNidec/1(CAN3_HVBatCnctReq_toNidec) -> [CAN3_HVBatCnctReq_toNidec]
  HVSysReadyToChargetoNidec/1(CAN3_HVSysReadyToCharge_toNidec) -> [CAN3_HVSysReadyToCharge_toNidec]
  LVChrgFuncStaChktoNidec/1(CAN3_LVChrgFuncStaChk_toNidec) -> [CAN3_LVChrgFuncStaChk_toNidec]
  MSACrlStatoNidec/1(CAN3_MSA_Crl_Sta_toNidec) -> [CAN3_MSA_Crl_Sta_toNidec]
  PrkReqtoNidec/1(CAN3_PrkReq_toNidec) -> [CAN3_PrkReq_toNidec]
  PwrStatoNidec/1(CAN3_PwrSta_toNidec) -> [CAN3_PwrSta_toNidec]
  RCVCU1toNidec/1(CAN3_RC_VCU1_toNidec) -> [CAN3_RC_VCU1_toNidec]
  RrActvDmpDisabReqtoNidec/1(CAN3_Rr_ActvDmpDisabReq_toNidec) -> [CAN3_Rr_ActvDmpDisabReq_toNidec]
  RrMCUEnaReqtoNidec/1(CAN3_Rr_MCUEnaReq_toNidec) -> [CAN3_Rr_MCUEnaReq_toNidec]
  ShiftGearPosntoNidec/1(CAN3_ShiftGearPosn_toNidec) -> [CAN3_ShiftGearPosn_toNidec]
  bus_selector/1 -> ActiveDischReqtoNidec/1(ActiveDischReqtoNidec)  "<VOUTP_ActiveDischargeReq_flg>"
  [BOUTP_outputs] -> bus_selector/1
  Ground/1 -> CSVCU1toNidec/1(CSVCU1toNidec)
  Ground1/1 -> CoastDwModeStaChktoNidec/1(CoastDwModeStaChktoNidec)
  bus_selector1/1 -> DCDCEnaReqtoNidec/1(DCDCEnaReqtoNidec)  "<VOUTP_DCDCEnaReq_flg>"
  [BOUTP_outputs] -> bus_selector1/1
  bus_selector2/1 -> DCDCVoltSetpointtoNidec/1(DCDCVoltSetpointtoNidec)  "<VOUTP_DCDCVoltSetpoint_V>"
  [BOUTP_outputs] -> bus_selector2/1
  Ground2/1 -> DemoModeStaChktoNidec/1(DemoModeStaChktoNidec)
  bus_selector3/1 -> DrSeatStatoNidec/1(DrSeatStatoNidec)  "<VOUTP_DrSeatSta_enum>"
  [BOUTP_outputs] -> bus_selector3/1
  Ground3/1 -> DynoModeStaChktoNidec/1(DynoModeStaChktoNidec)
  bus_selector4/1 -> FrActvDmpDisabReqtoNidec/1(FrActvDmpDisabReqtoNidec)  "<VOUTP_FrActvDmpDisabReq_flg>"
  [BOUTP_outputs] -> bus_selector4/1
  bus_selector5/1 -> FrMCUEnaReqtoNidec/1(FrMCUEnaReqtoNidec)  "<VOUTP_FrMCUEnaReq_flg>"
  [BOUTP_outputs] -> bus_selector5/1
  bus_selector6/1 -> HVBatCnctReqtoNidec/1(HVBatCnctReqtoNidec)  "<VOUTP_HVBatCnctReq_flg>"
  [BOUTP_outputs] -> bus_selector6/1
  bus_selector7/1 -> HVSysReadyToChargetoNidec/1(HVSysReadyToChargetoNidec)  "<VOUTP_HVSysReadyToCharge_enum>"
  [BOUTP_outputs] -> bus_selector7/1
  Ground4/1 -> LVChrgFuncStaChktoNidec/1(LVChrgFuncStaChktoNidec)
  bus_selector8/1 -> MSACrlStatoNidec/1(MSACrlStatoNidec)  "<VOUTP_MSACtrlSta_enum>"
  [BOUTP_outputs] -> bus_selector8/1
  bus_selector9/1 -> PrkReqtoNidec/1(PrkReqtoNidec)  "<VOUTP_ActParkRequest_flg>"
  [BOUTP_outputs] -> bus_selector9/1
  bus_selector10/1 -> PwrStatoNidec/1(PwrStatoNidec)  "<VOUTP_PowerSta_enum>"
  [BOUTP_outputs] -> bus_selector10/1
  Ground5/1 -> RCVCU1toNidec/1(RCVCU1toNidec)
  bus_selector11/1 -> RrActvDmpDisabReqtoNidec/1(RrActvDmpDisabReqtoNidec)  "<VOUTP_RrActvDmpDisabReq_flg>"
  [BOUTP_outputs] -> bus_selector11/1
  bus_selector12/1 -> RrMCUEnaReqtoNidec/1(RrMCUEnaReqtoNidec)  "<VOUTP_RrMCUEnaReq_flg>"
  [BOUTP_outputs] -> bus_selector12/1
  bus_selector13/1 -> ShiftGearPosntoNidec/1(ShiftGearPosntoNidec)  "<VOUTP_ShiftGearPosn_enum>"
  [BOUTP_outputs] -> bus_selector13/1

== system halout/HAL_OUT/CAN3/FD3_VCU1_toNIDEC_Tx ==
  TxReq : Inport
  BSCP_outputs : Inport  Port=2  OutDataTypeStr=Bus: BSCP_outputs
  BOUTP_outputs : Inport  Port=3  OutDataTypeStr=Bus: BOUTP_outputs
  Chart : Stateflow chart  TreatAsAtomicUnit=on
  Constant : Constant  Value=C_TASK_5MS_S
  Constant3 : Constant  Value=CycleTime
  Data Type Conversion : DataTypeConversion  OutDataTypeStr=uint16
  Data Type Conversion1 : DataTypeConversion  OutDataTypeStr=uint8
  Divide : Product  Inputs=*/
  Gain : Gain  Gain=0.001
  Ground{,1..5} (6 alike) : Ground
  OR : Logic  Operator=OR  Inputs=20  AllPortsSameDT=off  OutDataTypeStr=boolean
  bus_selector : BusSelector  OutputSignals=VOUTP_ActiveDischargeReq_flg
  bus_selector1 : BusSelector  OutputSignals=VOUTP_DCDCEnaReq_flg
  bus_selector10 : BusSelector  OutputSignals=VOUTP_PowerSta_enum
  bus_selector11 : BusSelector  OutputSignals=VOUTP_RrActvDmpDisabReq_flg
  bus_selector12 : BusSelector  OutputSignals=VOUTP_RrMCUEnaReq_flg
  bus_selector13 : BusSelector  OutputSignals=VOUTP_ShiftGearPosn_enum
  bus_selector2 : BusSelector  OutputSignals=VOUTP_DCDCVoltSetpoint_V
  bus_selector3 : BusSelector  OutputSignals=VOUTP_DrSeatSta_enum
  bus_selector4 : BusSelector  OutputSignals=VOUTP_FrActvDmpDisabReq_flg
  bus_selector5 : BusSelector  OutputSignals=VOUTP_FrMCUEnaReq_flg
  bus_selector6 : BusSelector  OutputSignals=VOUTP_HVBatCnctReq_flg
  bus_selector7 : BusSelector  OutputSignals=VOUTP_HVSysReadyToCharge_enum
  bus_selector8 : BusSelector  OutputSignals=VOUTP_MSACtrlSta_enum
  bus_selector9 : BusSelector  OutputSignals=VOUTP_ActParkRequest_flg
  convert_out : FVT_lib/hal/convert_out  gain=0.0235  offset=12
  detect_change{,1..13} (14 alike) : simulink/Logic and Bit Operations/Detect Change  vinit=0  OutDataTypeStr=boolean
  TxTrigger : Outport
  wires:
  Data Type Conversion/1 -> Chart/3(CycleCnt)
  TxReq/1 -> Chart/1(TxReq)
  [EventReq_flg] -> Chart/2(EventReq)
  Constant/1 -> Divide/2
  Divide/1 -> Data Type Conversion/1
  Chart/1(TxTrigger) -> TxTrigger/1
  Gain/1 -> Divide/1
  Constant3/1 -> Gain/1
  BSCP_outputs/1 -> [BSCP_outputs]
  BOUTP_outputs/1 -> [BOUTP_outputs]
  OR/1 -> [EventReq_flg]
  detect_change/1 -> OR/1
  bus_selector/1 -> detect_change/1  "<VOUTP_ActiveDischargeReq_flg>"
  [BOUTP_outputs] -> bus_selector/1
  Ground/1 -> OR/2
  Ground1/1 -> OR/3
  detect_change1/1 -> OR/4
  bus_selector1/1 -> detect_change1/1  "<VOUTP_DCDCEnaReq_flg>"
  [BOUTP_outputs] -> bus_selector1/1
  detect_change2/1 -> OR/5
  Data Type Conversion1/1 -> detect_change2/1
  convert_out/1 -> Data Type Conversion1/1
  bus_selector2/1 -> convert_out/1  "<VOUTP_DCDCVoltSetpoint_V>"
  [BOUTP_outputs] -> bus_selector2/1
  Ground2/1 -> OR/6
  detect_change3/1 -> OR/7
  bus_selector3/1 -> detect_change3/1  "<VOUTP_DrSeatSta_enum>"
  [BOUTP_outputs] -> bus_selector3/1
  Ground3/1 -> OR/8
  detect_change4/1 -> OR/9
  bus_selector4/1 -> detect_change4/1  "<VOUTP_FrActvDmpDisabReq_flg>"
  [BOUTP_outputs] -> bus_selector4/1
  detect_change5/1 -> OR/10
  bus_selector5/1 -> detect_change5/1  "<VOUTP_FrMCUEnaReq_flg>"
  [BOUTP_outputs] -> bus_selector5/1
  detect_change6/1 -> OR/11
  bus_selector6/1 -> detect_change6/1  "<VOUTP_HVBatCnctReq_flg>"
  [BOUTP_outputs] -> bus_selector6/1
  detect_change7/1 -> OR/12
  bus_selector7/1 -> detect_change7/1  "<VOUTP_HVSysReadyToCharge_enum>"
  [BOUTP_outputs] -> bus_selector7/1
  Ground4/1 -> OR/13
  detect_change8/1 -> OR/14
  bus_selector8/1 -> detect_change8/1  "<VOUTP_MSACtrlSta_enum>"
  [BOUTP_outputs] -> bus_selector8/1
  detect_change9/1 -> OR/15
  bus_selector9/1 -> detect_change9/1  "<VOUTP_ActParkRequest_flg>"
  [BOUTP_outputs] -> bus_selector9/1
  detect_change10/1 -> OR/16
  bus_selector10/1 -> detect_change10/1  "<VOUTP_PowerSta_enum>"
  [BOUTP_outputs] -> bus_selector10/1
  Ground5/1 -> OR/17
  detect_change11/1 -> OR/18
  bus_selector11/1 -> detect_change11/1  "<VOUTP_RrActvDmpDisabReq_flg>"
  [BOUTP_outputs] -> bus_selector11/1
  detect_change12/1 -> OR/19
  bus_selector12/1 -> detect_change12/1  "<VOUTP_RrMCUEnaReq_flg>"
  [BOUTP_outputs] -> bus_selector12/1
  detect_change13/1 -> OR/20
  bus_selector13/1 -> detect_change13/1  "<VOUTP_ShiftGearPosn_enum>"
  [BOUTP_outputs] -> bus_selector13/1
